simulink model "P"  (R2016b)
settings: Solver=FixedStepAuto  StartTime=0.0  StopTime=10.0  FixedStep=0.01  RelTol=1e-3
values from neighbouring files (symbols this model uses):
  den = [1 0.1313 1.109]    [UpdatedSimulinkValues-2.m]    (also in UpdatedSimulinkValuesalex1.m; part2a.m)
  num = [0.26*1.109*180/pi()]    [UpdatedSimulinkValues-2.m]    (also in UpdatedSimulinkValuesalex1.m; part2a.m)
undefined symbols (not defined in the file or in its folder): G
settings Model: Creator=Akash  LastModifiedBy=Alex
settings SolverCC: ZeroCrossAlgorithm=Adaptive

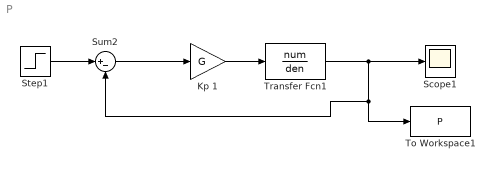
== system P ==
  Kp 1 : Gain  Gain=G
  Scope1 : Scope
  Step1 : Step  SampleTime=0
  Sum2 : Sum  Inputs=|+-
  To Workspace1 : ToWorkspace  VariableName=P  SaveFormat=Timeseries  SampleTime=-1
  Transfer Fcn1 : TransferFcn  Numerator=num  Denominator=den
  wires:
  Step1/1 -> Sum2/1
  Sum2/1 -> Kp 1/1
  Transfer Fcn1/1 -> Sum2/2, To Workspace1/1, Scope1/1
  Kp 1/1 -> Transfer Fcn1/1
